simulink model "titled"  (R2015b)
settings: Solver=VariableStepAuto  StartTime=0.0  StopTime=0.05  RelTol=1e-3
libraries: dspsrcs4 x2
settings Model: Creator=Lukas  LastModifiedBy=Lukas

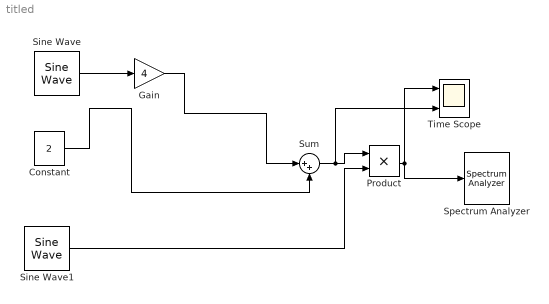
== system titled ==
  Constant : Constant  Value=2  VectorParams1D=off
  Gain : Gain  Gain=4
  Product : Product
  Sine Wave : dspsrcs4/Sine Wave  Amplitude=1  Frequency=100  Phase=0  SampleMode=Discrete  OutComplex=Real  CompMethod=Trigonometric fcn  TableSize=Speed  SampleTime=1/10000  SamplesPerFrame=1  ResetState=Restart at time zero  OutputFrames=off  dataType=double  wordLen=16  udDataType=sfix(16)  fracBitsMode=Best precision  numFracBits=15  OutDataTypeStr=double  LastOutDataTypeStr=double
  Sine Wave1 : dspsrcs4/Sine Wave  Amplitude=1  Frequency=1000  Phase=0  SampleMode=Discrete  OutComplex=Real  CompMethod=Trigonometric fcn  TableSize=Speed  SampleTime=1/10000  SamplesPerFrame=1  ResetState=Restart at time zero  OutputFrames=off  dataType=double  wordLen=16  udDataType=sfix(16)  fracBitsMode=Best precision  numFracBits=15  OutDataTypeStr=double  LastOutDataTypeStr=double
  Spectrum Analyzer : SpectrumAnalyzer
  Sum : Sum  Inputs=|++
  Time Scope : Scope  NumInputPorts=2
  wires:
  Sine Wave/1 -> Gain/1
  Constant/1 -> Sum/2
  Product/1 -> Time Scope/1, Spectrum Analyzer/1
  Sum/1 -> Time Scope/2, Product/1
  Sine Wave1/1 -> Product/2
  Gain/1 -> Sum/1
